simulink model "untitled1"  (R2019b)
settings: Solver=VariableStepAuto  StartTime=0.0  StopTime=10.0  RelTol=1e-3
libraries: neural x1015
(part 4 of 13)

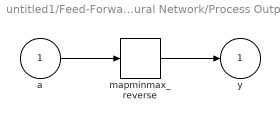
== system untitled1/Feed-Forward Neural Network/Process Output 1 ==
  a : Inport  PortDimensions=1001  SampleTime=0.1
      mask Display: e = 0.06;c1 = [120 230 180]/255;c2 = ([120 230 180]+0)/(256+128);c3 = ([120 230 180]+128)/(256+128);patch([0 1 1 0],[0 0 1 1],c1);patch([0 1 1 1-e 1-e 0+e],[0 0 1 1-e 0+e 0+e],c2);patch([0 0 1 1-e 0+e 0+e],[0 1 1 1-e 1-e 0+e],c3);plot([0 1 1 0 0],[0 0 1 1 0]);
  mapminmax_reverse : neural/Processing Functions/mapminmax_reverse  xmin=[-1.71317793350087788084579187853;-0.369716888993999459600559021055;0.985884072502071551191704656958;1.35682534104763297122531184868;1.1201718375194267274252979405;0.984869142682815112976868476835;0.920719873171212510598593325994;0.876451958923907481491255566652;0.828164621571482295614430313435;0.768139243071301991427901612042;0.695943029683275926622343376948;0.614697727350764000497918004839;0.529266624899904836176744993281;0.444890338602465740258651294425;0.366053305813792251299787494645;0.295790600263589054108592790726;0.2355453003982849735642446376;0.185443521157788226982887636041;0.14474196020984300692369117769;0.112251722753097984974779421918;0.0866485153554940046305432588269;0.0666603161744823147216720826691;0.0511601226094830774382415938817;0.0391975461224632198975470487312;0.0299963491706304180572928430593;0.0229359126546896628651150962241;0.0175271712331088250214072843391;0.0133885349830461658493518939395;0.0102243014384834074448349383601;0.00780640517508067108276570422731;0.00595952111715969141264581665496;0.0045491725066988328296524457528;0.00347237461032425800619427569416;0.00265034464652910781851113952712;0.00202285881043419695640706024165;0.00154390373092988053907448353641;0.00117833564646654346402820934259;0.000899319130589191031467655168541;0.00068636627454874918081301204964;0.000523837028200436431030206918535;0.000399793010081527910165588579616;0.000305121876055176421797809904746;0.000232868590866474570351407624713;0.000177724822949046020771624032619;0.000135639130652782436727010750843;0.00010351939451975705557516815869;7.90056817980926942741881635612e-05;6.02968804146319659878136554276e-05;4.60183777791158162007167931051e-05;3.51210691266955359383060419898e-05;2.68042786762646642346324954431e-05;2.0456932086077363219019792373e-05;1.56126588535713357527856537388e-05;1.19155262791259951185400545182e-05;9.0938875970777958306946742173e-06;6.94042285481137177088895029442e-06;5.29690614659686611806997669216e-06;4.04257999961077007583997930396e-06;3.08528272060097233451658044201e-06;2.35467682755490736754640408723e-06;1.79708099960965357158094481138e-06;1.37152584049370633267049025827e-06;1.04674365408801543989437791982e-06;7.98871041252380848703162387336e-07;6.09695544146118473195945786092e-07;4.65317473858375015039747727569e-07;3.55128642979857694023462528349e-07;2.71032920468411354009054953229e-07;2.06851363120358614326597035057e-07;1.57868226235915557360009811583e-07;1.20484468996568288410198462046e-07;9.19533196221755795333286731888e-08;7.01784463724631886813324146979e-08;5.3559941645036204880161014117e-08;4.08767584846377606134354681239e-08;3.1196997024790735704637839338e-08;2.38094362340344075795242064723e-08;1.81712772749398669639519203348e-08;1.38682548448194404640419880015e-08;1.05842020352130411718616625344e-08;8.07782531313363644388176915308e-09;6.16496801218116493761733134518e-09;4.70508019306507543785863791281e-09;3.59090152858720577712576742344e-09;2.74056337421489903267284229265e-09;2.09158823911702587829862410999e-09;1.59629277548361045369904322416e-09;1.21828456340643098982091586431e-09;9.29790403609544231745573747455e-10;7.09613821656852125212947757151e-10;5.41573898012393063980244200839e-10;4.1332776363541408098060982801e-10;3.15449802696896676260977716481e-10;2.40750820648745402297365457894e-10;1.83739517327695512104839397663e-10;1.40229055388737426259397040289e-10;1.07021756992896853519720292108e-10;8.16789044863661444140603637341e-11;6.23379760912086786833750951224e-11;4.75745263128377355945967171721e-11;3.6308711064269853586378585428e-11;2.77118127903781802213191104275e-11;2.11490394245251399572646018748e-11;1.61404602613847430566930969098e-11;1.23191515349664872972311187279e-11;9.401898323232067035471673285e-12;7.17524307410335740747807470966e-12;5.47734868927275541924448838988e-12;4.17846646061434086373638067786e-12;3.18930695457909307073032615933e-12;2.43453221161002494095754682641e-12;1.85973148313820255885872009287e-12;1.41746975759070798655828012935e-12 ...(+11489 chars)]  xmax=[1.7394902026542444772871931491;1.57211215723791286613675310946;1.54567524962036184632552249241;1.90423893338479244263794498693;2.30349876154407207096141974034;2.4446943461013805887205307954;2.52934387394229798218248106423;2.63286082209035621204407107143;2.77914185406077418605264028884;2.97515196155317696025122131687;3.22169287107719659601912098879;3.51704526267134198747044138145;3.85871785922696730608549842145;4.24467473754481616765588114504;4.67418777481569058807053806959;5.14821374991806202103816758608;5.66933891497068920273250114406;6.24148905964520039901799464133;6.86961098505333023211960608023;7.5594405600495298003238531237;8.31738202881270716204653581372;9.15047672005248990956260968233;10.0664296451110768515491145081;11.0736693642379542268372460967;12.1814263152455950489638780709;13.3998223095100357227238419;14.7399684367701748755052904016;16.2140709901134698611713247374;17.8355461298412194537377217785;19.6191444753475146001164830523;21.5810870038527866654476383701;23.73921372296887000175047433;26.1131466519366064460427878657;28.7244687268432343785207194742;31.596920349313410980585103971;34.7566154284989536904504348058;38.2322789222838750333721691277;42.0555080646963403978588758036;46.2610596722611902009703044314;50.8871661527976328898148494773;55.9758830969790892595483455807;61.5734716174163381197104172315;67.7308189141849368297698674724;74.5039008921186507450329372659;81.9542910367627115419963956811;90.1497201759555224498399184085;99.1646922163071877776019391604;109.081161452518145438261853997;119.989277607111773704673396423;131.988205373808398235269123688;145.187025915024207733949879184;159.705728508983781921415356919;175.676301361456495442325831391;193.243931498610862718123826198;212.56832464911821034547756426;233.825157114444152739451965317;257.207672826153782352776033804;282.928440108939184938208200037;311.221284119942083634668961167;342.343412532006027504394296557;376.577753785251388762844726443;414.235529163805097141448641196;455.659082080204029807646293193;501.224990288236199376115109771;551.347489317067243064229842275;606.482238248778799061255995184;667.130462073659828092786483467;733.843508281027766315673943609;807.227859109131827608507592231;887.950645020045840283273719251;976.745709522050901796319521964;1074.42028047425628756172955036;1181.86230852168228011578321457;1300.04853937385041717789135873;1430.05339331123559531988576055;1573.05873264235901842766907066;1730.3646059065949884825386107;1903.40106649725476017920300364;2093.74117314698014524765312672;2303.11529046167834167135879397;2533.42681950784617583849467337;2786.76950145863065699813887477;3065.44645160449363174848258495;3371.99109676494299492333084345;3709.19020644143711251672357321;4080.10922708558064186945557594;4488.12014979413834225852042437;4936.93216477355235838331282139;5430.62538125090759422164410353;5973.68791937599871744168922305;6571.05671131359849823638796806;7228.1623824449579842621460557;7950.97862068945414648624137044;8746.07648275839892448857426643;9620.68413103423881693743169308;10582.752544137661971035413444;11641.0277985514276224421337247;12805.1305784065698389895260334;14085.6436362472268228884786367;15494.2079998719491413794457912;17043.628799859143327921628952;18747.9916798450576607137918472;20622.7908478295648819766938686;22685.0699326125213701743632555;24953.5769258737745985854417086;27448.9346184611531498376280069;30193.8280803072702838107943535;33213.2108883379987673833966255;36534.5319771717986441217362881;40187.9851748889777809381484985;44206.7836923778741038404405117;48627.4620616156607866287231445;53490.208267777226865291595459;58839.2290945549466414377093315;64723.152004010444215964525938;71195.4672044114849995821714401;78315.0139248526393203064799309;86146.515317337907617911696434;94761.1668490716983797028660774;104237.283533978872583247721195;114661.011887376764207147061825;126127.113076114444993436336517;138739.824383725877851247787476;152613.80682209847145713865757;167875.187504308327334001660347 ...(+25362 chars)]  ymin=-1  ymax=1
      settings: SourceProductName=Deep Learning Toolbox
  y : Outport  PortDimensions=1001  SampleTime=0.1
      mask Display: e = 0.06;c1 = [120 230 180]/255;c2 = ([120 230 180]+0)/(256+128);c3 = ([120 230 180]+128)/(256+128);patch([0 1 1 0],[0 0 1 1],c1);patch([0 1 1 1-e 1-e 0+e],[0 0 1 1-e 0+e 0+e],c2);patch([0 0 1 1-e 0+e 0+e],[0 1 1 1-e 1-e 0+e],c3);plot([0 1 1 0 0],[0 0 1 1 0]);
  wires:
  a/1 -> mapminmax_reverse/1
  mapminmax_reverse/1 -> y/1

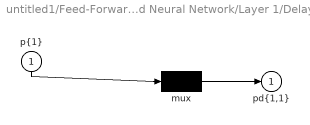
== system untitled1/Feed-Forward Neural Network/Layer 1/Delays 1 ==
  "p{1}" : Inport  PortDimensions=1001  SampleTime=0.1
      mask Display: e = 0.06;c1 = [120 230 180]/255;c2 = ([120 230 180]+0)/(256+128);c3 = ([120 230 180]+128)/(256+128);patch([0 1 1 0],[0 0 1 1],c1);patch([0 1 1 1-e 1-e 0+e],[0 0 1 1-e 0+e 0+e],c2);patch([0 0 1 1-e 0+e 0+e],[0 1 1 1-e 1-e 0+e],c3);plot([0 1 1 0 0],[0 0 1 1 0]);
  mux : Mux  Inputs=1
      mask Display: e = 0.06;c1 = [120 150 230]/255;c2 = ([120 150 230]+0)/383;c3 = ([120 150 230]+128)/383;patch([0 1 1 0],[0 0 1 1],c1);patch([0 1 1 1-e 1-e 0+e],[0 0 1 1-e 0+e 0+e],c2);patch([0 0 1 1-e 0+e 0+e],[0 1 1 1-e 1-e 0+e],c3);plot([0 1 1 0 0],[0 0 1 1 0]);disp('Mux')
  "pd{1,1}" : Outport
      mask Display: e = 0.06;c1 = [120 230 180]/255;c2 = ([120 230 180]+0)/(256+128);c3 = ([120 230 180]+128)/(256+128);patch([0 1 1 0],[0 0 1 1],c1);patch([0 1 1 1-e 1-e 0+e],[0 0 1 1-e 0+e 0+e],c2);patch([0 0 1 1-e 0+e 0+e],[0 1 1 1-e 1-e 0+e],c3);plot([0 1 1 0 0],[0 0 1 1 0]);
  wires:
  "p{1}"/1 -> mux/1
  mux/1 -> "pd{1,1}"/1
